simulink model "simulink_model"  (Simulink 8.0)
settings: Solver=ode45  StartTime=0.0  StopTime=1  RelTol=1e-3
libraries: simulink_need_slupdate x1
settings Model: Creator=benoit  LastModifiedBy=yjiang  ExtModeAutoUpdateStatusClock=off
settings DataIOCC: SignalLoggingSaveFormat=ModelDataLogs  SignalLoggingName=sigsOut
settings OptimizationCC: InitFltsAndDblsToZero=on
settings DebuggingCC: SaveWithParameterizedLinksMsg=none  SignalResolutionControl=TryResolveAllWithWarning  SolverPrmCheckMsg=none  MultiTaskDSMMsg=warning  MultiTaskCondExecSysMsg=none  FcnCallInpInsideContextMsg=UseLocalSettings  StrictBusMsg=None
settings HardwareCC: TargetUnknown=on
settings RTWCC: IncludeERTFirstTime=on
settings GRTTargetCC: TargetFcnLib=ansi_tfl_tmw.mat  CombineOutputUpdateFcns=off  GRTInterface=on

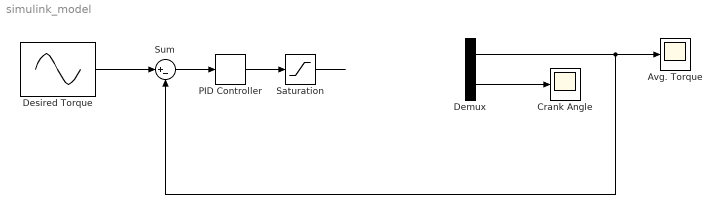
== system simulink_model ==
  Avg. Torque : Scope
      settings: TimeRange=1  YMin=-30  YMax=80
  Crank Angle : Scope
      settings: TimeRange=1.4  YMin=-200  YMax=800
  Demux : Demux  Outputs=2
  Desired Torque : Sin  Amplitude=20  Bias=50  Frequency=2  SampleTime=0
  PID Controller : simulink_need_slupdate/PID Controller  P=0.1  I=5  D=0
  Saturation : Saturate  UpperLimit=1000  LowerLimit=0
  Sum : Sum  Inputs=|+-  SaturateOnIntegerOverflow=on
  wires:
  ? -> Demux/1
  Demux/1 -> Sum/2, Avg. Torque/1
  Desired Torque/1 -> Sum/1
  Sum/1 -> PID Controller/1
  PID Controller/1 -> Saturation/1
  Demux/2 -> Crank Angle/1
  Saturation/1 -> ?
